simulink model "frac_test"  (Simulink 8.3)
settings: Solver=ode45  StartTime=0.0  StopTime=10.0  RelTol=1e-3
values from neighbouring files (symbols this model uses):
  FraOrder = CalFracPra( FraAlpha,n)    [initialization1.m]    (also in test_ousta_fod.m = CalFracPra(-0.5,4))
settings Model: Creator=wayne  LastModifiedBy=wayne
settings DataIOCC: ExternalInput=[t]  LimitDataPoints=off  SaveFormat=StructureWithTime  SignalLoggingSaveFormat=Dataset  TimeSaveName=t  OutputSaveName=y2
settings DebuggingCC: UnderspecifiedInitializationDetection=Simplified  StateNameClashWarn=none
settings GRTTargetCC: CombineOutputUpdateFcns=on  GRTInterface=off

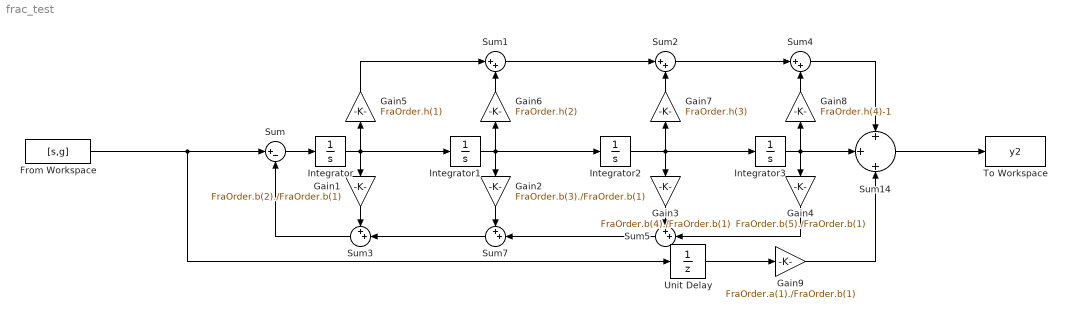
== system frac_test ==
  From Workspace : FromWorkspace  VariableName=[s,g]  SampleTime=0
  Gain1 : Gain  Gain=FraOrder.b(2)./FraOrder.b(1)
  Gain2 : Gain  Gain=FraOrder.b(3)./FraOrder.b(1)
  Gain3 : Gain  Gain=FraOrder.b(4)./FraOrder.b(1)
  Gain4 : Gain  Gain=FraOrder.b(5)./FraOrder.b(1)
  Gain5 : Gain  Gain=FraOrder.h(1)
  Gain6 : Gain  Gain=FraOrder.h(2)
  Gain7 : Gain  Gain=FraOrder.h(3)
  Gain8 : Gain  Gain=FraOrder.h(4)-1
  Gain9 : Gain  Gain=FraOrder.a(1)./FraOrder.b(1)
  Integrator{,1..3} (4 alike) : Integrator
  Sum : Sum  Inputs=|+-
  Sum1 : Sum  Inputs=|++
  Sum14 : Sum  Inputs=+||+||+
  Sum2 : Sum  Inputs=|++
  Sum3 : Sum  Inputs=++|
  Sum4 : Sum  Inputs=|++
  Sum5 : Sum  Inputs=++|
  Sum7 : Sum  Inputs=++|
  To Workspace : ToWorkspace  VariableName=y2  SaveFormat=Structure With Time  SampleTime=-1
  Unit Delay : UnitDelay  SampleTime=-1
  wires:
  Sum/1 -> Integrator/1
  Integrator/1 -> Gain5/1, Integrator1/1, Gain1/1
  Sum3/1 -> Sum/2
  Gain1/1 -> Sum3/1
  Integrator2/1 -> Gain7/1, Integrator3/1, Gain3/1
  Integrator3/1 -> Gain8/1, Gain4/1, Sum14/2
  Sum5/1 -> Sum7/2
  Gain3/1 -> Sum5/1
  Gain4/1 -> Sum5/2
  Integrator1/1 -> Gain6/1, Integrator2/1, Gain2/1
  Sum7/1 -> Sum3/2
  Gain2/1 -> Sum7/1
  Sum14/1 -> To Workspace/1
  Unit Delay/1 -> Gain9/1
  Gain5/1 -> Sum1/1
  Gain6/1 -> Sum1/2
  Sum1/1 -> Sum2/1
  Gain7/1 -> Sum2/2
  Sum2/1 -> Sum4/1
  Gain8/1 -> Sum4/2
  Sum4/1 -> Sum14/1
  Gain9/1 -> Sum14/3
  From Workspace/1 -> Unit Delay/1, Sum/1
